simulink model "Prim_Sim_12B_qvt"  (R2012b)
settings: Solver=FixedStepDiscrete  StartTime=0.0  StopTime=500  FixedStep=0.1  RelTol=1e-3
libraries: simulink x14
settings Model: Creator=Kerianne  LastModifiedBy=jonathan
settings DataIOCC: SignalLoggingSaveFormat=ModelDataLogs  SignalLogging=off
settings OptimizationCC: InlineParams=on
settings DebuggingCC: MultiTaskDSMMsg=warning  MultiTaskCondExecSysMsg=none
settings RTWCC: IncludeERTFirstTime=on
settings CodeAppCC: CustomSymbolStrType=$N$R$M_T
settings GRTTargetCC: CodeReplacementLibrary=C89/C90 (ANSI)

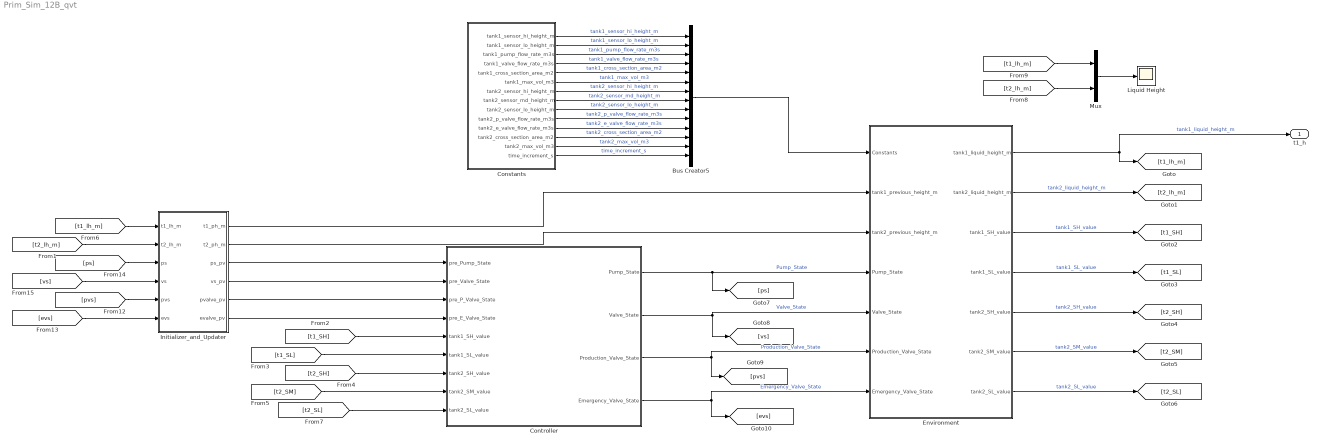
== system Prim_Sim_12B_qvt ==
  Bus Creator5 : BusCreator  Inputs=14
  Constants : Subsystem
  Controller : Subsystem
  Environment : Subsystem
  Initializer_and_Updater : Subsystem
  Liquid Height : Scope
  Mux : Mux  Inputs=2
  t1_h : Outport
  wires:
  Environment/1(tank1_liquid_height_m) -> [t1_lh_m], t1_h/1  "tank1_liquid_height_m"
  Environment/2(tank2_liquid_height_m) -> [t2_lh_m]  "tank2_liquid_height_m"
  Initializer_and_Updater/1(t1_ph_m) -> Environment/2(tank1_previous_height_m)
  Initializer_and_Updater/2(t2_ph_m) -> Environment/3(tank2_previous_height_m)
  Environment/3(tank1_SH_value) -> [t1_SH]  "tank1_SH_value"
  Environment/4(tank1_SL_value) -> [t1_SL]  "tank1_SL_value"
  Environment/5(tank2_SH_value) -> [t2_SH]  "tank2_SH_value"
  Environment/6(tank2_SM_value) -> [t2_SM]  "tank2_SM_value"
  Environment/7(tank2_SL_value) -> [t2_SL]  "tank2_SL_value"
  Initializer_and_Updater/6(evalve_pv) -> Controller/4(pre_E_Valve_State)
  Initializer_and_Updater/3(ps_pv) -> Controller/1(pre_Pump_State)
  Initializer_and_Updater/4(vs_pv) -> Controller/2(pre_Valve_State)
  Initializer_and_Updater/5(pvalve_pv) -> Controller/3(pre_P_Valve_State)
  [t1_SH] -> Controller/5(tank1_SH_value)
  [t1_SL] -> Controller/6(tank1_SL_value)
  [t2_SH] -> Controller/7(tank2_SH_value)
  [t2_SM] -> Controller/8(tank2_SM_value)
  [t2_SL] -> Controller/9(tank2_SL_value)
  Constants/1(tank1_sensor_hi_height_m) -> Bus Creator5/1  "tank1_sensor_hi_height_m"
  Constants/10(tank2_p_valve_flow_rate_m3s) -> Bus Creator5/10  "tank2_p_valve_flow_rate_m3s"
  Constants/9(tank2_sensor_lo_height_m) -> Bus Creator5/9  "tank2_sensor_lo_height_m"
  Constants/12(tank2_cross_section_area_m2) -> Bus Creator5/12  "tank2_cross_section_area_m2"
  Constants/11(tank2_e_valve_flow_rate_m3s) -> Bus Creator5/11  "tank2_e_valve_flow_rate_m3s"
  Constants/4(tank1_valve_flow_rate_m3s) -> Bus Creator5/4  "tank1_valve_flow_rate_m3s"
  Constants/2(tank1_sensor_lo_height_m) -> Bus Creator5/2  "tank1_sensor_lo_height_m"
  Constants/3(tank1_pump_flow_rate_m3s) -> Bus Creator5/3  "tank1_pump_flow_rate_m3s"
  Constants/6(tank1_max_vol_m3) -> Bus Creator5/6  "tank1_max_vol_m3"
  Constants/7(tank2_sensor_hi_height_m) -> Bus Creator5/7  "tank2_sensor_hi_height_m"
  Constants/8(tank2_sensor_md_height_m) -> Bus Creator5/8  "tank2_sensor_md_height_m"
  Constants/5(tank1_cross_section_area_m2) -> Bus Creator5/5  "tank1_cross_section_area_m2"
  Constants/13(tank2_max_vol_m3) -> Bus Creator5/13  "tank2_max_vol_m3"
  Bus Creator5/1 -> Environment/1(Constants)
  Constants/14(time_increment_s) -> Bus Creator5/14  "time_increment_s"
  [t1_lh_m] -> Initializer_and_Updater/1(t1_lh_m)
  [t2_lh_m] -> Initializer_and_Updater/2(t2_lh_m)
  Controller/1(Pump_State) -> Environment/4(Pump_State), [ps]  "Pump_State"
  Controller/2(Valve_State) -> Environment/5(Valve_State), [vs]  "Valve_State"
  Controller/3(Production_Valve_State) -> [pvs], Environment/6(Production_Valve_State)  "Production_Valve_State"
  Controller/4(Emergency_Valve_State) -> [evs], Environment/7(Emergency_Valve_State)  "Emergency_Valve_State"
  [ps] -> Initializer_and_Updater/3(ps)
  [vs] -> Initializer_and_Updater/4(vs)
  [pvs] -> Initializer_and_Updater/5(pvs)
  [evs] -> Initializer_and_Updater/6(evs)
  [t1_lh_m] -> Mux/1
  [t2_lh_m] -> Mux/2
  Mux/1 -> Liquid Height/1

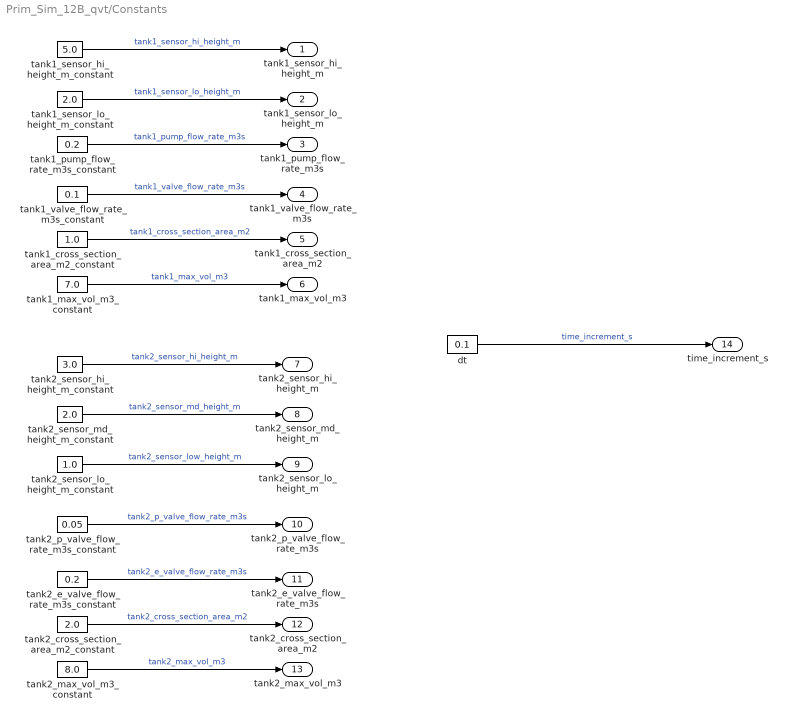
== system Prim_Sim_12B_qvt/Constants ==
  dt : Constant  Value=0.1
  tank1_cross_section_area_m2_constant : Constant  Value=1.0
  tank1_max_vol_m3_constant : Constant  Value=7.0
  tank1_pump_flow_rate_m3s_constant : Constant  Value=0.2
  tank1_sensor_hi_height_m_constant : Constant  Value=5.0
  tank1_sensor_lo_height_m_constant : Constant  Value=2.0
  tank1_valve_flow_rate_m3s_constant : Constant  Value=0.1
  tank2_cross_section_area_m2_constant : Constant  Value=2.0
  tank2_e_valve_flow_rate_m3s_constant : Constant  Value=0.2
  tank2_max_vol_m3_constant : Constant  Value=8.0
  tank2_p_valve_flow_rate_m3s_constant : Constant  Value=0.05
  tank2_sensor_hi_height_m_constant : Constant  Value=3.0
  tank2_sensor_lo_height_m_constant : Constant  Value=1.0
  tank2_sensor_md_height_m_constant : Constant  Value=2.0
  tank1_sensor_hi_height_m : Outport
  tank1_sensor_lo_height_m : Outport  Port=2
  tank1_pump_flow_rate_m3s : Outport  Port=3
  tank1_valve_flow_rate_m3s : Outport  Port=4
  tank1_cross_section_area_m2 : Outport  Port=5
  tank1_max_vol_m3 : Outport  Port=6
  tank2_sensor_hi_height_m : Outport  Port=7
  tank2_sensor_md_height_m : Outport  Port=8
  tank2_sensor_lo_height_m : Outport  Port=9
  tank2_p_valve_flow_rate_m3s : Outport  Port=10
  tank2_e_valve_flow_rate_m3s : Outport  Port=11
  tank2_cross_section_area_m2 : Outport  Port=12
  tank2_max_vol_m3 : Outport  Port=13
  time_increment_s : Outport  Port=14
  wires:
  tank2_sensor_hi_height_m_constant/1 -> tank2_sensor_hi_height_m/1  "tank2_sensor_hi_height_m"
  tank2_sensor_lo_height_m_constant/1 -> tank2_sensor_lo_height_m/1  "tank2_sensor_low_height_m"
  tank1_sensor_hi_height_m_constant/1 -> tank1_sensor_hi_height_m/1  "tank1_sensor_hi_height_m"
  tank1_pump_flow_rate_m3s_constant/1 -> tank1_pump_flow_rate_m3s/1  "tank1_pump_flow_rate_m3s"
  tank1_cross_section_area_m2_constant/1 -> tank1_cross_section_area_m2/1  "tank1_cross_section_area_m2"
  tank1_valve_flow_rate_m3s_constant/1 -> tank1_valve_flow_rate_m3s/1  "tank1_valve_flow_rate_m3s"
  tank1_sensor_lo_height_m_constant/1 -> tank1_sensor_lo_height_m/1  "tank1_sensor_lo_height_m"
  tank2_p_valve_flow_rate_m3s_constant/1 -> tank2_p_valve_flow_rate_m3s/1  "tank2_p_valve_flow_rate_m3s"
  tank2_e_valve_flow_rate_m3s_constant/1 -> tank2_e_valve_flow_rate_m3s/1  "tank2_e_valve_flow_rate_m3s"
  tank2_sensor_md_height_m_constant/1 -> tank2_sensor_md_height_m/1  "tank2_sensor_md_height_m"
  tank1_max_vol_m3_constant/1 -> tank1_max_vol_m3/1  "tank1_max_vol_m3"
  tank2_cross_section_area_m2_constant/1 -> tank2_cross_section_area_m2/1  "tank2_cross_section_area_m2"
  tank2_max_vol_m3_constant/1 -> tank2_max_vol_m3/1  "tank2_max_vol_m3"
  dt/1 -> time_increment_s/1  "time_increment_s"

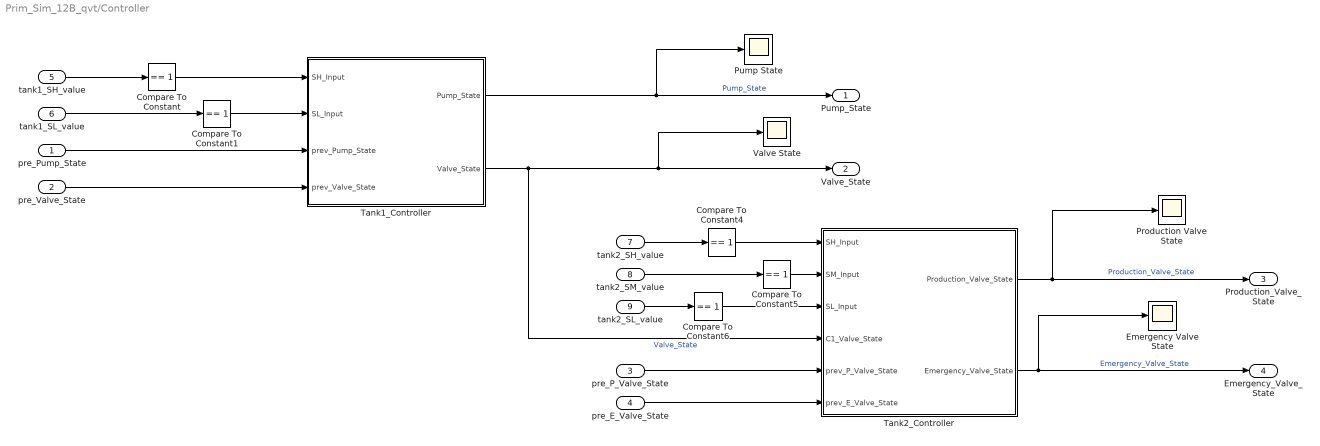
== system Prim_Sim_12B_qvt/Controller ==
  pre_Pump_State : Inport
  pre_Valve_State : Inport  Port=2
  pre_P_Valve_State : Inport  Port=3
  pre_E_Valve_State : Inport  Port=4
  tank1_SH_value : Inport  Port=5
  tank1_SL_value : Inport  Port=6
  tank2_SH_value : Inport  Port=7
  tank2_SM_value : Inport  Port=8
  tank2_SL_value : Inport  Port=9
  Compare To Constant{,1,4..6} (5 alike) : simulink/Logic and Bit Operations/Compare To Constant  relop===  const=1  OutDataTypeStr=boolean
  Emergency Valve State : Scope
      settings: SaveName=ScopeData3
  Production Valve State : Scope
      settings: SaveName=ScopeData2
  "Pump State " : Scope
      settings: SaveName=ScopeData4
  Tank1_Controller : Subsystem
  Tank2_Controller : Subsystem
  Valve State : Scope
  Pump_State : Outport
  Valve_State : Outport  Port=2
  Production_Valve_State : Outport  Port=3
  Emergency_Valve_State : Outport  Port=4
  wires:
  tank1_SL_value/1 -> Compare To Constant1/1
  tank2_SL_value/1 -> Compare To Constant6/1
  pre_E_Valve_State/1 -> Tank2_Controller/6(prev_E_Valve_State)
  Compare To Constant1/1 -> Tank1_Controller/2(SL_Input)
  Tank1_Controller/1(Pump_State) -> Pump_State/1, "Pump State "/1  "Pump_State"
  Tank1_Controller/2(Valve_State) -> Tank2_Controller/4(C1_Valve_State), Valve_State/1, Valve State/1  "Valve_State"
  Compare To Constant/1 -> Tank1_Controller/1(SH_Input)
  pre_Pump_State/1 -> Tank1_Controller/3(prev_Pump_State)
  tank2_SH_value/1 -> Compare To Constant4/1
  Compare To Constant6/1 -> Tank2_Controller/3(SL_Input)
  Compare To Constant4/1 -> Tank2_Controller/1(SH_Input)
  tank1_SH_value/1 -> Compare To Constant/1
  pre_Valve_State/1 -> Tank1_Controller/4(prev_Valve_State)
  Tank2_Controller/2(Emergency_Valve_State) -> Emergency_Valve_State/1, Emergency Valve State/1  "Emergency_Valve_State"
  tank2_SM_value/1 -> Compare To Constant5/1
  Compare To Constant5/1 -> Tank2_Controller/2(SM_Input)
  Tank2_Controller/1(Production_Valve_State) -> Production_Valve_State/1, Production Valve State/1  "Production_Valve_State"
  pre_P_Valve_State/1 -> Tank2_Controller/5(prev_P_Valve_State)

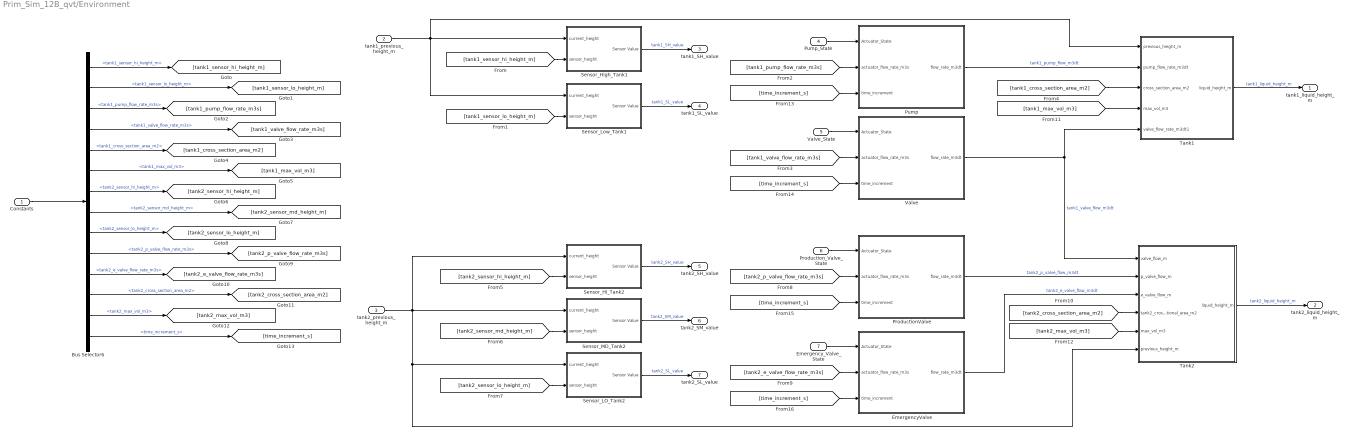
== system Prim_Sim_12B_qvt/Environment ==
  Constants : Inport
  tank1_previous_height_m : Inport  Port=2
  tank2_previous_height_m : Inport  Port=3
  Pump_State : Inport  Port=4
  Valve_State : Inport  Port=5
  Production_Valve_State : Inport  Port=6
  Emergency_Valve_State : Inport  Port=7
  Bus Selector6 : BusSelector  OutputSignals=tank1_sensor_hi_height_m,tank1_sensor_lo_height_m,tank1_pump_flow_rate_m3s,tank1_valve_flow_rate_m3s,tank1_cross_section_area_m2,tank1_max_vol_m3,tank2_sensor_hi_height_m,tank2_sensor_md_height_m,tank2_sensor_lo_height_m,tank2_p_valve_flow_rate_m3s,tank2_e_valve_flow_rate_m3s,tank2_cross_section_area_m2,tank2_max_vol_m3,time_increment_s
  EmergencyValve : Subsystem
  ProductionValve : Subsystem
  Pump : Subsystem
  Sensor_HI_Tank2 : Subsystem
  Sensor_High_Tank1 : Subsystem
  Sensor_LO_Tank2 : Subsystem
  Sensor_Low_Tank1 : Subsystem
  Sensor_MD_Tank2 : Subsystem
  Tank1 : Subsystem
  Tank2 : Subsystem
  Valve : Subsystem
  tank1_liquid_height_m : Outport
  tank2_liquid_height_m : Outport  Port=2
  tank1_SH_value : Outport  Port=3
  tank1_SL_value : Outport  Port=4
  tank2_SH_value : Outport  Port=5
  tank2_SM_value : Outport  Port=6
  tank2_SL_value : Outport  Port=7
  wires:
  Tank1/1(liquid_height_m) -> tank1_liquid_height_m/1  "tank1_liquid_height_m"
  [tank2_sensor_hi_height_m] -> Sensor_HI_Tank2/2(sensor_height)
  [tank2_sensor_md_height_m] -> Sensor_MD_Tank2/2(sensor_height)
  Sensor_Low_Tank1/1(Sensor Value) -> tank1_SL_value/1  "tank1_SL_value"
  Sensor_HI_Tank2/1(Sensor Value) -> tank2_SH_value/1  "tank2_SH_value"
  Sensor_High_Tank1/1(Sensor Value) -> tank1_SH_value/1  "tank1_SH_value"
  [tank1_pump_flow_rate_m3s] -> Pump/2(actuator_flow_rate_m3s)
  Sensor_LO_Tank2/1(Sensor Value) -> tank2_SL_value/1  "tank2_SL_value"
  [tank2_sensor_lo_height_m] -> Sensor_LO_Tank2/2(sensor_height)
  [tank1_valve_flow_rate_m3s] -> Valve/2(actuator_flow_rate_m3s)
  Sensor_MD_Tank2/1(Sensor Value) -> tank2_SM_value/1  "tank2_SM_value"
  tank2_previous_height_m/1 -> Sensor_LO_Tank2/1(current_height), Tank2/6(previous_height_m), Sensor_MD_Tank2/1(current_height), Sensor_HI_Tank2/1(current_height)
  EmergencyValve/1(flow_rate_m3dt) -> Tank2/3(e_valve_flow_m)  "tank2_e_valve_flow_m3dt"
  Pump/1(flow_rate_m3dt) -> Tank1/2(pump_flow_rate_m3dt)  "tank1_pump_flow_m3dt"
  Valve/1(flow_rate_m3dt) -> Tank2/1(valve_flow_m), Tank1/5(valve_flow_rate_m3dt1)  "tank1_valve_flow_m3dt"
  ProductionValve/1(flow_rate_m3dt) -> Tank2/2(p_valve_flow_m)  "tank2_p_valve_flow_m3dt"
  [tank2_e_valve_flow_rate_m3s] -> EmergencyValve/2(actuator_flow_rate_m3s)
  Valve_State/1 -> Valve/1(Actuator_State)
  Emergency_Valve_State/1 -> EmergencyValve/1(Actuator_State)
  Pump_State/1 -> Pump/1(Actuator_State)
  Production_Valve_State/1 -> ProductionValve/1(Actuator_State)
  tank1_previous_height_m/1 -> Tank1/1(previous_height_m), Sensor_Low_Tank1/1(current_height), Sensor_High_Tank1/1(current_height)
  Tank2/1(liquid_height_m) -> tank2_liquid_height_m/1  "tank2_liquid_height_m"
  [tank1_cross_section_area_m2] -> Tank1/3(cross_section_area_m2)
  [tank2_cross_section_area_m2] -> Tank2/4(tank2_cross_sectional_area_m2)
  Bus Selector6/1 -> [tank1_sensor_hi_height_m]  "<tank1_sensor_hi_height_m>"
  [tank1_sensor_hi_height_m] -> Sensor_High_Tank1/2(sensor_height)
  Constants/1 -> Bus Selector6/1
  Bus Selector6/2 -> [tank1_sensor_lo_height_m]  "<tank1_sensor_lo_height_m>"
  Bus Selector6/3 -> [tank1_pump_flow_rate_m3s]  "<tank1_pump_flow_rate_m3s>"
  [tank1_sensor_lo_height_m] -> Sensor_Low_Tank1/2(sensor_height)
  Bus Selector6/4 -> [tank1_valve_flow_rate_m3s]  "<tank1_valve_flow_rate_m3s>"
  Bus Selector6/5 -> [tank1_cross_section_area_m2]  "<tank1_cross_section_area_m2>"
  Bus Selector6/6 -> [tank1_max_vol_m3]  "<tank1_max_vol_m3>"
  Bus Selector6/7 -> [tank2_sensor_hi_height_m]  "<tank2_sensor_hi_height_m>"
  Bus Selector6/8 -> [tank2_sensor_md_height_m]  "<tank2_sensor_md_height_m>"
  Bus Selector6/9 -> [tank2_sensor_lo_height_m]  "<tank2_sensor_lo_height_m>"
  Bus Selector6/10 -> [tank2_p_valve_flow_rate_m3s]  "<tank2_p_valve_flow_rate_m3s>"
  Bus Selector6/11 -> [tank2_e_valve_flow_rate_m3s]  "<tank2_e_valve_flow_rate_m3s>"
  [tank2_p_valve_flow_rate_m3s] -> ProductionValve/2(actuator_flow_rate_m3s)
  Bus Selector6/12 -> [tank2_cross_section_area_m2]  "<tank2_cross_section_area_m2>"
  Bus Selector6/13 -> [tank2_max_vol_m3]  "<tank2_max_vol_m3>"
  [tank1_max_vol_m3] -> Tank1/4(max_vol_m3)
  [tank2_max_vol_m3] -> Tank2/5(max_vol_m3)
  Bus Selector6/14 -> [time_increment_s]  "<time_increment_s>"
  [time_increment_s] -> Pump/3(time_increment)
  [time_increment_s] -> Valve/3(time_increment)
  [time_increment_s] -> ProductionValve/3(time_increment)
  [time_increment_s] -> EmergencyValve/3(time_increment)

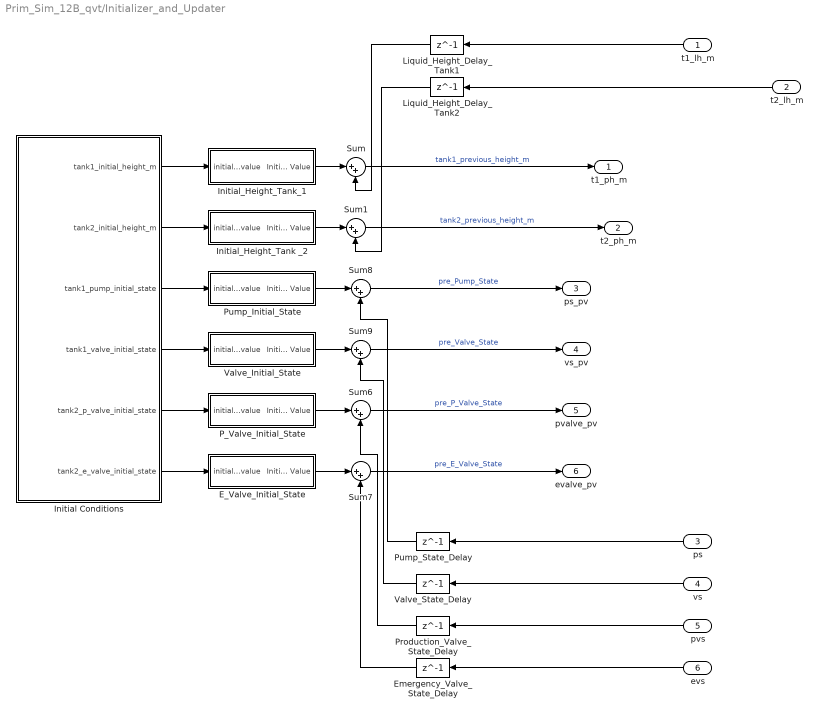
== system Prim_Sim_12B_qvt/Initializer_and_Updater ==
  t1_lh_m : Inport
  t2_lh_m : Inport  Port=2
  ps : Inport  Port=3
  vs : Inport  Port=4
  pvs : Inport  Port=5
  evs : Inport  Port=6
  E_Valve_Initial_State : Subsystem
  Emergency_Valve_State_Delay : Delay  DelayLength=1  InitialCondition=0
  Initial Conditions : Subsystem
  Initial_Height_Tank _2 : Subsystem
  Initial_Height_Tank_1 : Subsystem
  Liquid_Height_Delay_Tank1 : Delay  DelayLength=1  InitialCondition=0
  Liquid_Height_Delay_Tank2 : Delay  DelayLength=1  InitialCondition=0
  P_Valve_Initial_State : Subsystem
  Production_Valve_State_Delay : Delay  DelayLength=1  InitialCondition=0
  Pump_Initial_State : Subsystem
  Pump_State_Delay : Delay  DelayLength=1  InitialCondition=0
  Sum{,1,6..9} (6 alike) : Sum  Inputs=|++
  Valve_Initial_State : Subsystem
  Valve_State_Delay : Delay  DelayLength=1  InitialCondition=0
  t1_ph_m : Outport
  t2_ph_m : Outport  Port=2
  ps_pv : Outport  Port=3
  vs_pv : Outport  Port=4
  pvalve_pv : Outport  Port=5
  evalve_pv : Outport  Port=6
  wires:
  Production_Valve_State_Delay/1 -> Sum6/2
  Liquid_Height_Delay_Tank1/1 -> Sum/2
  Pump_Initial_State/1(Initial Value) -> Sum8/1
  Liquid_Height_Delay_Tank2/1 -> Sum1/2
  Valve_Initial_State/1(Initial Value) -> Sum9/1
  E_Valve_Initial_State/1(Initial Value) -> Sum7/1
  Emergency_Valve_State_Delay/1 -> Sum7/2
  pvs/1 -> Production_Valve_State_Delay/1
  ps/1 -> Pump_State_Delay/1
  vs/1 -> Valve_State_Delay/1
  evs/1 -> Emergency_Valve_State_Delay/1
  Initial_Height_Tank _2/1(Initial Value) -> Sum1/1
  Initial_Height_Tank_1/1(Initial Value) -> Sum/1
  Initial Conditions/3(tank1_pump_initial_state) -> Pump_Initial_State/1(initial_value)
  Initial Conditions/4(tank1_valve_initial_state) -> Valve_Initial_State/1(initial_value)
  Initial Conditions/1(tank1_initial_height_m) -> Initial_Height_Tank_1/1(initial_value)
  Initial Conditions/2(tank2_initial_height_m) -> Initial_Height_Tank _2/1(initial_value)
  Initial Conditions/5(tank2_p_valve_initial_state) -> P_Valve_Initial_State/1(initial_value)
  Initial Conditions/6(tank2_e_valve_initial_state) -> E_Valve_Initial_State/1(initial_value)
  P_Valve_Initial_State/1(Initial Value) -> Sum6/1
  Sum7/1 -> evalve_pv/1  "pre_E_Valve_State"
  t2_lh_m/1 -> Liquid_Height_Delay_Tank2/1
  t1_lh_m/1 -> Liquid_Height_Delay_Tank1/1
  Sum6/1 -> pvalve_pv/1  "pre_P_Valve_State"
  Sum/1 -> t1_ph_m/1  "tank1_previous_height_m"
  Sum9/1 -> vs_pv/1  "pre_Valve_State"
  Sum8/1 -> ps_pv/1  "pre_Pump_State"
  Sum1/1 -> t2_ph_m/1  "tank2_previous_height_m"
  Valve_State_Delay/1 -> Sum9/2
  Pump_State_Delay/1 -> Sum8/2

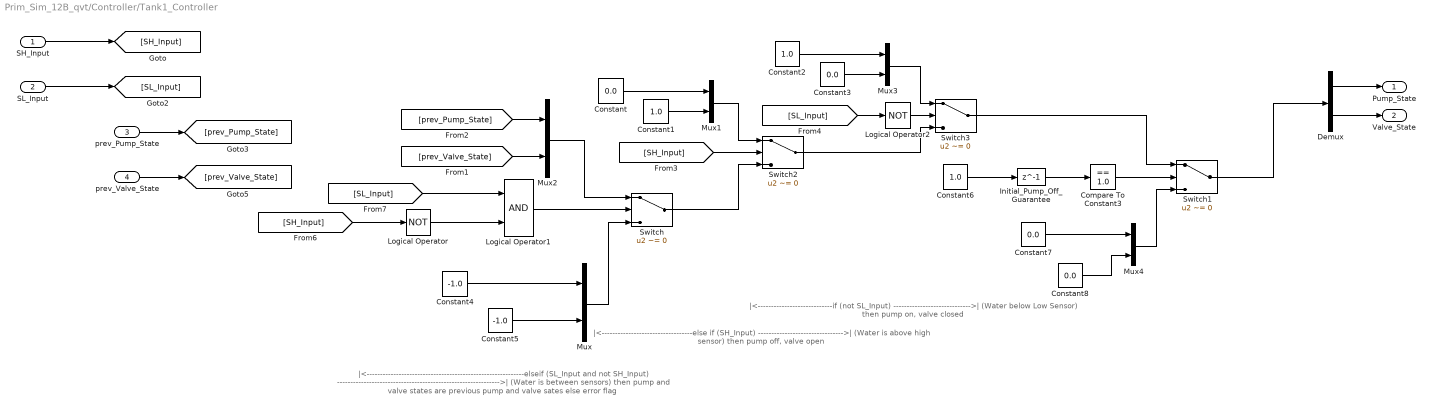
== system Prim_Sim_12B_qvt/Controller/Tank1_Controller ==
  note: |<----------------------------if (not SL_Input) ----------------------------->|
      | (Water below Low Sensor)
      | then pump on, valve closed
  note: |<----------------------------------else if (SH_Input) -------------------------------->|
      | (Water is above high sensor)
      | then pump off, valve open
  note: |<-----------------------------------------------------------elseif (SL_Input and not SH_Input) ------------------------------------------------------------->|
      | (Water is between sensors)
      | then pump and valve states are previous pump and valve sates
      | else error flag
  SH_Input : Inport
  SL_Input : Inport  Port=2
  prev_Pump_State : Inport  Port=3
  prev_Valve_State : Inport  Port=4
  Compare To Constant3 : simulink/Logic and Bit Operations/Compare To Constant  relop===  const=1.0  OutDataTypeStr=boolean
  Constant{,3,7..8} (4 alike) : Constant  Value=0.0
  Constant1 : Constant  Value=1.0
  Constant2 : Constant  Value=1.0
  Constant4 : Constant  Value=-1.0
  Constant5 : Constant  Value=-1.0
  Constant6 : Constant  Value=1.0
  Demux : Demux  Outputs=2
  Initial_Pump_Off_Guarantee : Delay  DelayLength=1
  Logical Operator : Logic  Operator=NOT  AllPortsSameDT=off  OutDataTypeStr=boolean
  Logical Operator1 : Logic  AllPortsSameDT=off  OutDataTypeStr=boolean
  Logical Operator2 : Logic  Operator=NOT  AllPortsSameDT=off  OutDataTypeStr=boolean
  Mux{,1..4} (5 alike) : Mux  Inputs=2
  Switch{,1..3} (4 alike) : Switch  Criteria=u2 ~= 0
  Pump_State : Outport
  Valve_State : Outport  Port=2
  wires:
  prev_Pump_State/1 -> [prev_Pump_State]
  prev_Valve_State/1 -> [prev_Valve_State]
  Mux/1 -> Switch/3
  Constant/1 -> Mux1/1
  Constant1/1 -> Mux1/2
  [prev_Pump_State] -> Mux2/1
  [prev_Valve_State] -> Mux2/2
  Mux2/1 -> Switch/1
  Logical Operator1/1 -> Switch/2
  [SL_Input] -> Logical Operator1/1
  Logical Operator/1 -> Logical Operator1/2
  [SH_Input] -> Logical Operator/1
  Switch/1 -> Switch2/3
  [SH_Input] -> Switch2/2
  Mux1/1 -> Switch2/1
  [SL_Input] -> Logical Operator2/1
  Constant2/1 -> Mux3/1
  Constant3/1 -> Mux3/2
  Mux3/1 -> Switch3/1
  Demux/2 -> Valve_State/1
  SH_Input/1 -> [SH_Input]
  SL_Input/1 -> [SL_Input]
  Logical Operator2/1 -> Switch3/2
  Constant4/1 -> Mux/1
  Constant5/1 -> Mux/2
  Demux/1 -> Pump_State/1
  Switch2/1 -> Switch3/3
  Constant6/1 -> Initial_Pump_Off_Guarantee/1
  Initial_Pump_Off_Guarantee/1 -> Compare To Constant3/1
  Compare To Constant3/1 -> Switch1/2
  Constant7/1 -> Mux4/1
  Constant8/1 -> Mux4/2
  Switch1/1 -> Demux/1
  Mux4/1 -> Switch1/3
  Switch3/1 -> Switch1/1

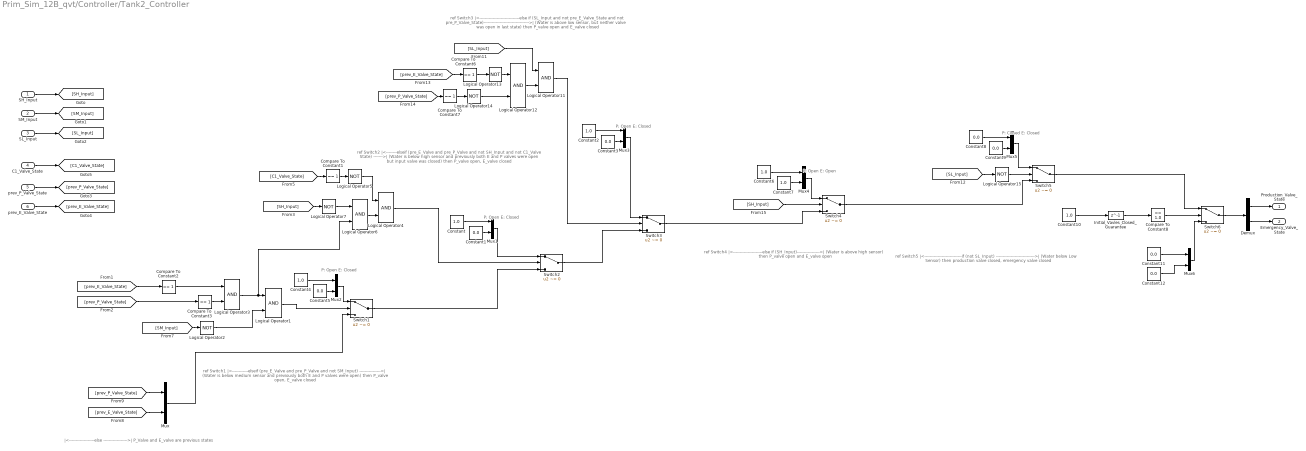
== system Prim_Sim_12B_qvt/Controller/Tank2_Controller ==
  note: P: Open
      | E: Closed
  note: P: Open
      | E: Closed
  note: P: Open
      | E: Closed
  note: P: Open
      | E: Open
  note: P: Closed
      | E: Closed
  note: ref Switch5
      | |<----------------------------if (not SL_Input) ----------------------------->|
      | (Water below Low Sensor)
      | then production valve closed, emergency valve closed
  note: ref Switch3
      | |<------------------------------else if (SL_Input and not pre_E_Valve_State and not pre_P_Valve_State)---------------------------------->|
      | (Water is above low sensor, but neither valve was open in last state)
      | then P_valve open and E_valve closed
  note: ref Switch2
      | |<--------elseif (pre_E_Valve and pre_P_Valve and not SH_Input and not C1_Valve State) ------->|
      | (Water is below high sensor  and previously both E and P valves were open but input valve was closed)
      | then P_valve open, E_valve closed
  note: ref Switch4
      | |<----------------------else if (SH_Input)----------------->|
      | (Water is above high sensor)
      | then P_valve open and E_valve open
  note: ref Switch1
      | |<------------elseif (pre_E_Valve and pre_P_Valve and not SM_Input) ---------------->|
      | (Water is below medium sensor and previously both E and P valves were open)
      | then P_valve open, E_valve closed
  note: |<-------------------else ------------------>|
      | P_Valve and E_valve are previous states
  SH_Input : Inport
  SM_Input : Inport  Port=2
  SL_Input : Inport  Port=3
  C1_Valve_State : Inport  Port=4
  prev_P_Valve_State : Inport  Port=5
  prev_E_Valve_State : Inport  Port=6
  Compare To Constant{1..3,6..7} (5 alike) : simulink/Logic and Bit Operations/Compare To Constant  relop===  const=1  OutDataTypeStr=boolean
  Compare To Constant8 : simulink/Logic and Bit Operations/Compare To Constant  relop===  const=1.0  OutDataTypeStr=boolean
  Constant{,2,4,6..7,10} (6 alike) : Constant  Value=1.0
  Constant{1,3,5,8..9,11..12} (7 alike) : Constant  Value=0.0
  Demux : Demux  Outputs=2
  Initial_Vavles_Closed_Guarantee : Delay  DelayLength=1
  Logical Operator{1,3..4,6,11..12} (6 alike) : Logic  AllPortsSameDT=off  OutDataTypeStr=boolean
  Logical Operator{2,5,7,13..15} (6 alike) : Logic  Operator=NOT  AllPortsSameDT=off  OutDataTypeStr=boolean
  Mux{,1..6} (7 alike) : Mux  Inputs=2
  Switch{1..6} (6 alike) : Switch  Criteria=u2 ~= 0
  Production_Valve_State : Outport
  Emergency_Valve_State : Outport  Port=2
  wires:
  SH_Input/1 -> [SH_Input]
  SL_Input/1 -> [SL_Input]
  SM_Input/1 -> [SM_Input]
  prev_E_Valve_State/1 -> [prev_E_Valve_State]
  C1_Valve_State/1 -> [C1_Valve_State]
  prev_P_Valve_State/1 -> [prev_P_Valve_State]
  [prev_P_Valve_State] -> Mux/1
  [prev_E_Valve_State] -> Mux/2
  Mux/1 -> Switch1/3
  Constant/1 -> Mux1/1
  Constant1/1 -> Mux1/2
  Logical Operator1/1 -> Switch1/2
  [SM_Input] -> Logical Operator2/1
  Switch1/1 -> Switch2/3
  Logical Operator4/1 -> Switch2/2
  Mux1/1 -> Switch2/1
  Demux/1 -> Production_Valve_State/1
  Demux/2 -> Emergency_Valve_State/1
  [prev_E_Valve_State] -> Compare To Constant2/1
  [prev_P_Valve_State] -> Compare To Constant3/1
  [C1_Valve_State] -> Compare To Constant1/1
  Logical Operator5/1 -> Logical Operator4/1
  Logical Operator6/1 -> Logical Operator4/2
  Logical Operator3/1 -> Logical Operator6/2, Logical Operator1/1
  Logical Operator2/1 -> Logical Operator1/2
  [SH_Input] -> Logical Operator7/1
  Logical Operator7/1 -> Logical Operator6/1
  Constant4/1 -> Mux2/1
  Constant5/1 -> Mux2/2
  Mux2/1 -> Switch1/1
  Constant2/1 -> Mux3/1
  Constant3/1 -> Mux3/2
  Mux3/1 -> Switch3/1
  [prev_E_Valve_State] -> Compare To Constant6/1
  [prev_P_Valve_State] -> Compare To Constant7/1
  Logical Operator13/1 -> Logical Operator12/1
  Logical Operator12/1 -> Logical Operator11/2
  [SL_Input] -> Logical Operator11/1
  Logical Operator14/1 -> Logical Operator12/2
  Constant6/1 -> Mux4/1
  Constant7/1 -> Mux4/2
  Mux4/1 -> Switch4/1
  Logical Operator15/1 -> Switch5/2
  [SL_Input] -> Logical Operator15/1
  Constant8/1 -> Mux5/1
  Constant9/1 -> Mux5/2
  Mux5/1 -> Switch5/1
  Compare To Constant1/1 -> Logical Operator5/1
  Compare To Constant2/1 -> Logical Operator3/1
  Compare To Constant3/1 -> Logical Operator3/2
  Compare To Constant6/1 -> Logical Operator13/1
  Compare To Constant7/1 -> Logical Operator14/1
  Constant10/1 -> Initial_Vavles_Closed_Guarantee/1
  Initial_Vavles_Closed_Guarantee/1 -> Compare To Constant8/1
  Compare To Constant8/1 -> Switch6/2
  Constant11/1 -> Mux6/1
  Constant12/1 -> Mux6/2
  Switch5/1 -> Switch6/1
  Mux6/1 -> Switch6/3
  Switch6/1 -> Demux/1
  [SH_Input] -> Switch4/2
  Logical Operator11/1 -> Switch3/2
  Switch2/1 -> Switch3/3
  Switch3/1 -> Switch4/3
  Switch4/1 -> Switch5/3

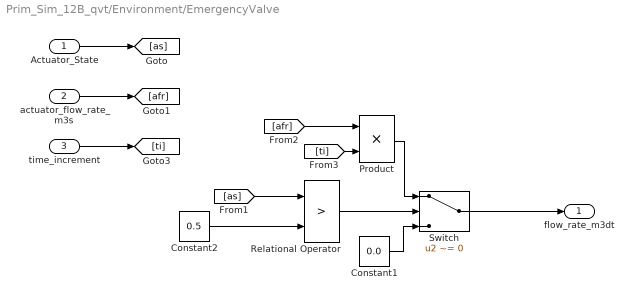
== system Prim_Sim_12B_qvt/Environment/EmergencyValve ==
  Actuator_State : Inport
  actuator_flow_rate_m3s : Inport  Port=2
  time_increment : Inport  Port=3
  Constant1 : Constant  Value=0.0
  Constant2 : Constant  Value=0.5
  Product : Product
  Relational Operator : RelationalOperator  Operator=>  OutDataTypeStr=boolean
  Switch : Switch  Criteria=u2 ~= 0
  flow_rate_m3dt : Outport
  wires:
  Relational Operator/1 -> Switch/2
  [as] -> Relational Operator/1
  [ti] -> Product/2
  Constant1/1 -> Switch/3
  Constant2/1 -> Relational Operator/2
  Actuator_State/1 -> [as]
  actuator_flow_rate_m3s/1 -> [afr]
  Switch/1 -> flow_rate_m3dt/1
  Product/1 -> Switch/1
  time_increment/1 -> [ti]
  [afr] -> Product/1

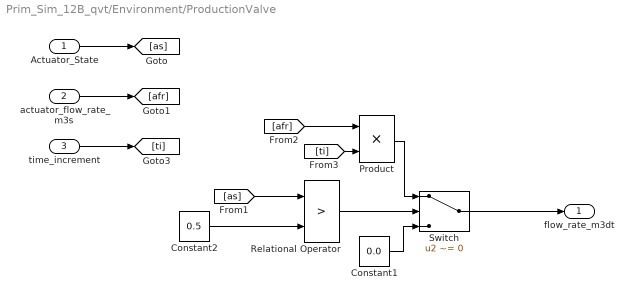
== system Prim_Sim_12B_qvt/Environment/ProductionValve ==
  Actuator_State : Inport
  actuator_flow_rate_m3s : Inport  Port=2
  time_increment : Inport  Port=3
  Constant1 : Constant  Value=0.0
  Constant2 : Constant  Value=0.5
  Product : Product
  Relational Operator : RelationalOperator  Operator=>  OutDataTypeStr=boolean
  Switch : Switch  Criteria=u2 ~= 0
  flow_rate_m3dt : Outport
  wires:
  [afr] -> Product/1
  time_increment/1 -> [ti]
  Product/1 -> Switch/1
  Switch/1 -> flow_rate_m3dt/1
  actuator_flow_rate_m3s/1 -> [afr]
  Actuator_State/1 -> [as]
  Constant2/1 -> Relational Operator/2
  Constant1/1 -> Switch/3
  [ti] -> Product/2
  [as] -> Relational Operator/1
  Relational Operator/1 -> Switch/2

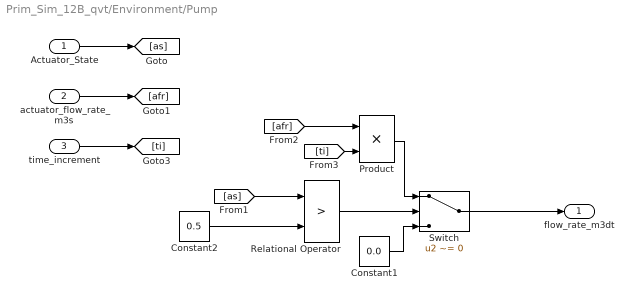
== system Prim_Sim_12B_qvt/Environment/Pump ==
  Actuator_State : Inport
  actuator_flow_rate_m3s : Inport  Port=2
  time_increment : Inport  Port=3
  Constant1 : Constant  Value=0.0
  Constant2 : Constant  Value=0.5
  Product : Product
  Relational Operator : RelationalOperator  Operator=>  OutDataTypeStr=boolean
  Switch : Switch  Criteria=u2 ~= 0
  flow_rate_m3dt : Outport
  wires:
  [afr] -> Product/1
  time_increment/1 -> [ti]
  Product/1 -> Switch/1
  Switch/1 -> flow_rate_m3dt/1
  actuator_flow_rate_m3s/1 -> [afr]
  Actuator_State/1 -> [as]
  Constant2/1 -> Relational Operator/2
  Constant1/1 -> Switch/3
  [ti] -> Product/2
  [as] -> Relational Operator/1
  Relational Operator/1 -> Switch/2

== system Prim_Sim_12B_qvt/Environment/Sensor_HI_Tank2 ==
  current_height : Inport
  sensor_height : Inport  Port=2
  Constant : Constant  Value=0.0
  Constant1 : Constant  Value=1.0
  Relational Operator : RelationalOperator  Operator=>  OutDataTypeStr=boolean
  Switch : Switch  Criteria=u2 ~= 0
  Sensor Value : Outport
  wires:
  Constant/1 -> Switch/1
  sensor_height/1 -> [sh]
  [sh] -> Relational Operator/1
  Constant1/1 -> Switch/3
  Relational Operator/1 -> Switch/2
  current_height/1 -> [ch]
  [ch] -> Relational Operator/2
  Switch/1 -> Sensor Value/1

== system Prim_Sim_12B_qvt/Environment/Sensor_High_Tank1 ==
  current_height : Inport
  sensor_height : Inport  Port=2
  Constant : Constant  Value=0.0
  Constant1 : Constant  Value=1.0
  Relational Operator : RelationalOperator  Operator=>  OutDataTypeStr=boolean
  Switch : Switch  Criteria=u2 ~= 0
  Sensor Value : Outport
  wires:
  Constant/1 -> Switch/1
  sensor_height/1 -> [sh]
  [sh] -> Relational Operator/1
  Constant1/1 -> Switch/3
  Relational Operator/1 -> Switch/2
  current_height/1 -> [ch]
  [ch] -> Relational Operator/2
  Switch/1 -> Sensor Value/1

== system Prim_Sim_12B_qvt/Environment/Sensor_LO_Tank2 ==
  current_height : Inport
  sensor_height : Inport  Port=2
  Constant : Constant  Value=0.0
  Constant1 : Constant  Value=1.0
  Relational Operator : RelationalOperator  Operator=>  OutDataTypeStr=boolean
  Switch : Switch  Criteria=u2 ~= 0
  Sensor Value : Outport
  wires:
  Constant/1 -> Switch/1
  sensor_height/1 -> [sh]
  [sh] -> Relational Operator/1
  Constant1/1 -> Switch/3
  Relational Operator/1 -> Switch/2
  current_height/1 -> [ch]
  [ch] -> Relational Operator/2
  Switch/1 -> Sensor Value/1

== system Prim_Sim_12B_qvt/Environment/Sensor_Low_Tank1 ==
  current_height : Inport
  sensor_height : Inport  Port=2
  Constant : Constant  Value=0.0
  Constant1 : Constant  Value=1.0
  Relational Operator : RelationalOperator  Operator=>  OutDataTypeStr=boolean
  Switch : Switch  Criteria=u2 ~= 0
  Sensor Value : Outport
  wires:
  Switch/1 -> Sensor Value/1
  [ch] -> Relational Operator/2
  current_height/1 -> [ch]
  Relational Operator/1 -> Switch/2
  Constant1/1 -> Switch/3
  [sh] -> Relational Operator/1
  sensor_height/1 -> [sh]
  Constant/1 -> Switch/1

== system Prim_Sim_12B_qvt/Environment/Sensor_MD_Tank2 ==
  current_height : Inport
  sensor_height : Inport  Port=2
  Constant : Constant  Value=0.0
  Constant1 : Constant  Value=1.0
  Relational Operator : RelationalOperator  Operator=>  OutDataTypeStr=boolean
  Switch : Switch  Criteria=u2 ~= 0
  Sensor Value : Outport
  wires:
  Switch/1 -> Sensor Value/1
  [ch] -> Relational Operator/2
  current_height/1 -> [ch]
  Relational Operator/1 -> Switch/2
  Constant1/1 -> Switch/3
  [sh] -> Relational Operator/1
  sensor_height/1 -> [sh]
  Constant/1 -> Switch/1

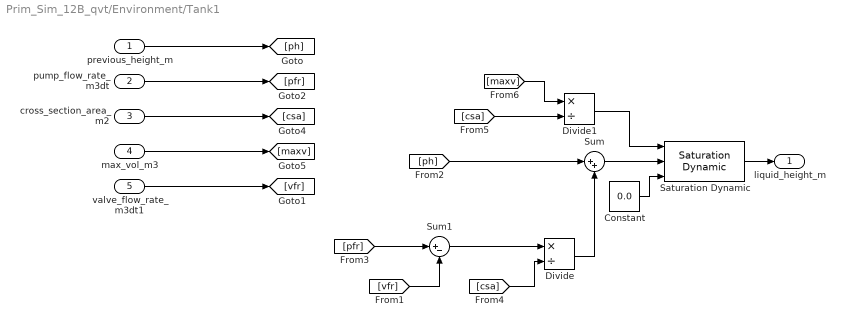
== system Prim_Sim_12B_qvt/Environment/Tank1 ==
  previous_height_m : Inport
  pump_flow_rate_m3dt : Inport  Port=2
  cross_section_area_m2 : Inport  Port=3
  max_vol_m3 : Inport  Port=4
  valve_flow_rate_m3dt1 : Inport  Port=5
  Constant : Constant  Value=0.0
  Divide : Product  Inputs=*/
  Divide1 : Product  Inputs=*/
  Saturation Dynamic : simulink/Discontinuities/Saturation Dynamic  OutMin=[]  OutMax=[]  OutDataTypeStr=Inherit: Same as second input  OutDataType=fixdt(1, 16)  OutScaling=2^-10  DoSatur=off
  Sum : Sum  Inputs=|++
  Sum1 : Sum  Inputs=|+-
  liquid_height_m : Outport
  wires:
  cross_section_area_m2/1 -> [csa]
  [ph] -> Sum/1
  Divide/1 -> Sum/2
  max_vol_m3/1 -> [maxv]
  [csa] -> Divide/2
  Sum1/1 -> Divide/1
  previous_height_m/1 -> [ph]
  [vfr] -> Sum1/2
  pump_flow_rate_m3dt/1 -> [pfr]
  [pfr] -> Sum1/1
  Saturation Dynamic/1 -> liquid_height_m/1
  Sum/1 -> Saturation Dynamic/2
  Constant/1 -> Saturation Dynamic/3
  valve_flow_rate_m3dt1/1 -> [vfr]
  Divide1/1 -> Saturation Dynamic/1
  [csa] -> Divide1/2
  [maxv] -> Divide1/1

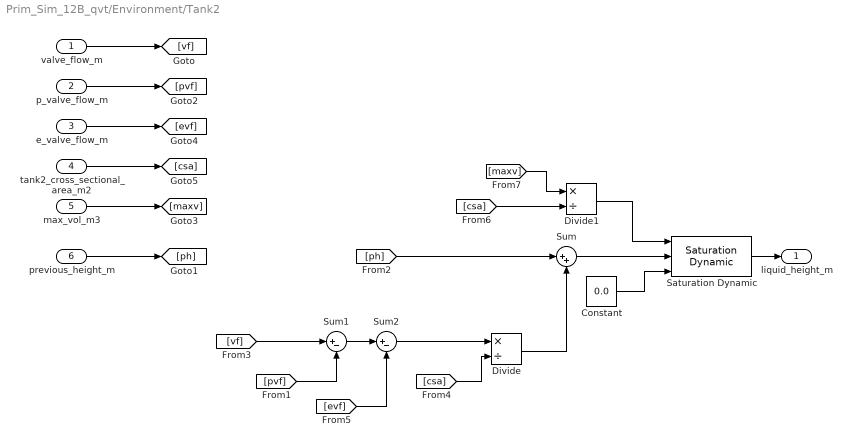
== system Prim_Sim_12B_qvt/Environment/Tank2 ==
  valve_flow_m : Inport
  p_valve_flow_m : Inport  Port=2
  e_valve_flow_m : Inport  Port=3
  tank2_cross_sectional_area_m2 : Inport  Port=4
  max_vol_m3 : Inport  Port=5
  previous_height_m : Inport  Port=6
  Constant : Constant  Value=0.0
  Divide : Product  Inputs=*/
  Divide1 : Product  Inputs=*/
  Saturation Dynamic : simulink/Discontinuities/Saturation Dynamic  OutMin=[]  OutMax=[]  OutDataTypeStr=Inherit: Same as second input  OutDataType=fixdt(1, 16)  OutScaling=2^-10  DoSatur=off
  Sum : Sum  Inputs=|++
  Sum1 : Sum  Inputs=|+-
  Sum2 : Sum  Inputs=|+-
  liquid_height_m : Outport
  wires:
  [evf] -> Sum2/2
  valve_flow_m/1 -> [vf]
  p_valve_flow_m/1 -> [pvf]
  Divide/1 -> Sum/2
  [csa] -> Divide/2
  [ph] -> Sum/1
  tank2_cross_sectional_area_m2/1 -> [csa]
  previous_height_m/1 -> [ph]
  [vf] -> Sum1/1
  e_valve_flow_m/1 -> [evf]
  Sum2/1 -> Divide/1
  [pvf] -> Sum1/2
  Sum1/1 -> Sum2/1
  max_vol_m3/1 -> [maxv]
  Saturation Dynamic/1 -> liquid_height_m/1
  Divide1/1 -> Saturation Dynamic/1
  Sum/1 -> Saturation Dynamic/2
  Constant/1 -> Saturation Dynamic/3
  [csa] -> Divide1/2
  [maxv] -> Divide1/1

== system Prim_Sim_12B_qvt/Environment/Valve ==
  Actuator_State : Inport
  actuator_flow_rate_m3s : Inport  Port=2
  time_increment : Inport  Port=3
  Constant1 : Constant  Value=0.0
  Constant2 : Constant  Value=0.5
  Product : Product
  Relational Operator : RelationalOperator  Operator=>  OutDataTypeStr=boolean
  Switch : Switch  Criteria=u2 ~= 0
  flow_rate_m3dt : Outport
  wires:
  Relational Operator/1 -> Switch/2
  [as] -> Relational Operator/1
  [ti] -> Product/2
  Constant1/1 -> Switch/3
  Constant2/1 -> Relational Operator/2
  Actuator_State/1 -> [as]
  actuator_flow_rate_m3s/1 -> [afr]
  Switch/1 -> flow_rate_m3dt/1
  Product/1 -> Switch/1
  time_increment/1 -> [ti]
  [afr] -> Product/1

== system Prim_Sim_12B_qvt/Initializer_and_Updater/E_Valve_Initial_State ==
  initial_value : Inport
  Constant : Constant  Value=0.0
  Switch : Switch  Criteria=u2 > Threshold
  Unit Delay : UnitDelay  InitialCondition=1  SampleTime=-1
  Initial Value : Outport
  wires:
  Switch/1 -> Initial Value/1
  Constant/1 -> Switch/3, Unit Delay/1
  Unit Delay/1 -> Switch/2
  initial_value/1 -> Switch/1

== system Prim_Sim_12B_qvt/Initializer_and_Updater/Initial Conditions ==
  tank1_init_height_m : Constant  Value=0.0
  tank1_pump_init_state : Constant  Value=0.0
  tank1_valve_init_state : Constant  Value=0.0
  tank2_e_valve_init_state : Constant  Value=0.0
  tank2_init_height_m : Constant  Value=0.0
  tank2_p_valve_init_state : Constant  Value=0.0
  tank1_initial_height_m : Outport
  tank2_initial_height_m : Outport  Port=2
  tank1_pump_initial_state : Outport  Port=3
  tank1_valve_initial_state : Outport  Port=4
  tank2_p_valve_initial_state : Outport  Port=5
  tank2_e_valve_initial_state : Outport  Port=6
  wires:
  tank1_pump_init_state/1 -> tank1_pump_initial_state/1  "tank1_pump_initial_state"
  tank2_e_valve_init_state/1 -> tank2_e_valve_initial_state/1  "tank2_e_valve_initial_state"
  tank2_p_valve_init_state/1 -> tank2_p_valve_initial_state/1  "tank2_p_valve_initial_state"
  tank1_init_height_m/1 -> tank1_initial_height_m/1  "tank1_initial_height_m"
  tank2_init_height_m/1 -> tank2_initial_height_m/1  "tank2_initial_height_m"
  tank1_valve_init_state/1 -> tank1_valve_initial_state/1  "tank1_valve_initial_state"

== system Prim_Sim_12B_qvt/Initializer_and_Updater/Initial_Height_Tank _2 ==
  initial_value : Inport
  Constant : Constant  Value=0.0
  Switch : Switch  Criteria=u2 > Threshold
  Unit Delay : UnitDelay  InitialCondition=1  SampleTime=-1
  Initial Value : Outport
  wires:
  Switch/1 -> Initial Value/1
  Constant/1 -> Switch/3, Unit Delay/1
  Unit Delay/1 -> Switch/2
  initial_value/1 -> Switch/1

== system Prim_Sim_12B_qvt/Initializer_and_Updater/Initial_Height_Tank_1 ==
  initial_value : Inport
  Constant : Constant  Value=0.0
  Switch : Switch  Criteria=u2 > Threshold
  Unit Delay : UnitDelay  InitialCondition=1  SampleTime=-1
  Initial Value : Outport
  wires:
  Switch/1 -> Initial Value/1
  Constant/1 -> Switch/3, Unit Delay/1
  Unit Delay/1 -> Switch/2
  initial_value/1 -> Switch/1

== system Prim_Sim_12B_qvt/Initializer_and_Updater/P_Valve_Initial_State ==
  initial_value : Inport
  Constant : Constant  Value=0.0
  Switch : Switch  Criteria=u2 > Threshold
  Unit Delay : UnitDelay  InitialCondition=1  SampleTime=-1
  Initial Value : Outport
  wires:
  Switch/1 -> Initial Value/1
  Constant/1 -> Switch/3, Unit Delay/1
  Unit Delay/1 -> Switch/2
  initial_value/1 -> Switch/1

== system Prim_Sim_12B_qvt/Initializer_and_Updater/Pump_Initial_State ==
  initial_value : Inport
  Constant : Constant  Value=0.0
  Switch : Switch  Criteria=u2 > Threshold
  Unit Delay : UnitDelay  InitialCondition=1  SampleTime=-1
  Initial Value : Outport
  wires:
  Switch/1 -> Initial Value/1
  Constant/1 -> Switch/3, Unit Delay/1
  Unit Delay/1 -> Switch/2
  initial_value/1 -> Switch/1

== system Prim_Sim_12B_qvt/Initializer_and_Updater/Valve_Initial_State ==
  initial_value : Inport
  Constant : Constant  Value=0.0
  Switch : Switch  Criteria=u2 > Threshold
  Unit Delay : UnitDelay  InitialCondition=1  SampleTime=-1
  Initial Value : Outport
  wires:
  Switch/1 -> Initial Value/1
  Constant/1 -> Switch/3, Unit Delay/1
  Unit Delay/1 -> Switch/2
  initial_value/1 -> Switch/1
